simulink model "UAVIntegratedNavigationSystem"  (R2020b)
settings: Solver=FixedStepAuto  StartTime=0.0  StopTime=TFinal  FixedStep=IMUtime  RelTol=1e-3
values from neighbouring files (symbols this model uses):
  AIONtime = 1    [ModelSettings.m]
  BiasAccel = 9.81E-4    (= 0.000981)    [ModelSettings.m]
  BiasGyro = 2.424068405548E-4    (= 0.000242406840555)    [ModelSettings.m]
  CorrTimeOrientationGNSS = 1    [ModelSettings.m]
  CorrTimePositionGNSS = 1    [ModelSettings.m]
  CorrTimeVelocityGNSS = 1    [ModelSettings.m]
  delay = 1.5    [ModelSettings.m]
  e = 0.081819106    [ModelSettings.m]
  g0 = 9.780327    [ModelSettings.m]
  GNSStime = 0.2    [ModelSettings.m]
  H0 = 0.1    [ModelSettings.m]
  IMUtime = 0.01    [ModelSettings.m]
  indUAV = 2    [ModelSettings.m]
  LambdaInit = 0.6555    [ModelSettings.m]
  mass = 0.7    [ModelSettings.m]
  N = 100    [ModelSettings.m]
  PhiInit = 0.968    [ModelSettings.m]
  PitchDown = -PitchUp    (= -0.1)    [ModelSettings.m]
  PitchUp = 0.1    [ModelSettings.m]
  Ra = 6378.245    [ModelSettings.m]
  RollDown = -RollUp    (= -0.1)    [ModelSettings.m]
  RollUp = 0.1    [ModelSettings.m]
  SigmaAccel = 9.81E-4    (= 0.000981)    [ModelSettings.m]
  SigmaAION = 30    [ModelSettings.m]
  SigmaAltitudeGNSS = 3    [ModelSettings.m]
  SigmaGyro = 2.666475246102E-6    (= 2.6664752461e-06)    [ModelSettings.m]
  SigmaLaser = 5    [ModelSettings.m]
  SigmaOrientationGNSS = 0.00349    [ModelSettings.m]
  SigmaPositionGNSS = 1.5    [ModelSettings.m]
  SigmaVelocityGNSS = 0.03    [ModelSettings.m]
  SigmaVelocityUpGNSS = 0.03    [ModelSettings.m]
  U1down = 0    [ModelSettings.m]
  U1up = 4 * ForceCoeff * OmegaMax^2    (= 9.9858124)    [ModelSettings.m]
  U2down = -U2up    (= -2.4964531)    [ModelSettings.m]
  U2up = ForceCoeff * OmegaMax^2    (= 2.4964531)    [ModelSettings.m]
  U3down = -U3up    (= -2.4964531)    [ModelSettings.m]
  U3up = ForceCoeff * OmegaMax^2    (= 2.4964531)    [ModelSettings.m]
  U4down = -U4up    (= -0.2494604)    [ModelSettings.m]
  U4up = 2 * DragCoeff * OmegaMax^2    (= 0.2494604)    [ModelSettings.m]
  WEarth = 7.2921158553E-5    (= 7.2921158553e-05)    [ModelSettings.m]
undefined symbols (not defined in the file or in its folder): deg, Newton, rad, Raphson, s
libraries: simulink x11, sharedtransform x7, pid_lib x6, aerolibconvert2 x4, sharedutil x4
(part 1 of 5)
settings Model: Creator=Павел Ермаков  LastModifiedBy=Павел Ермаков

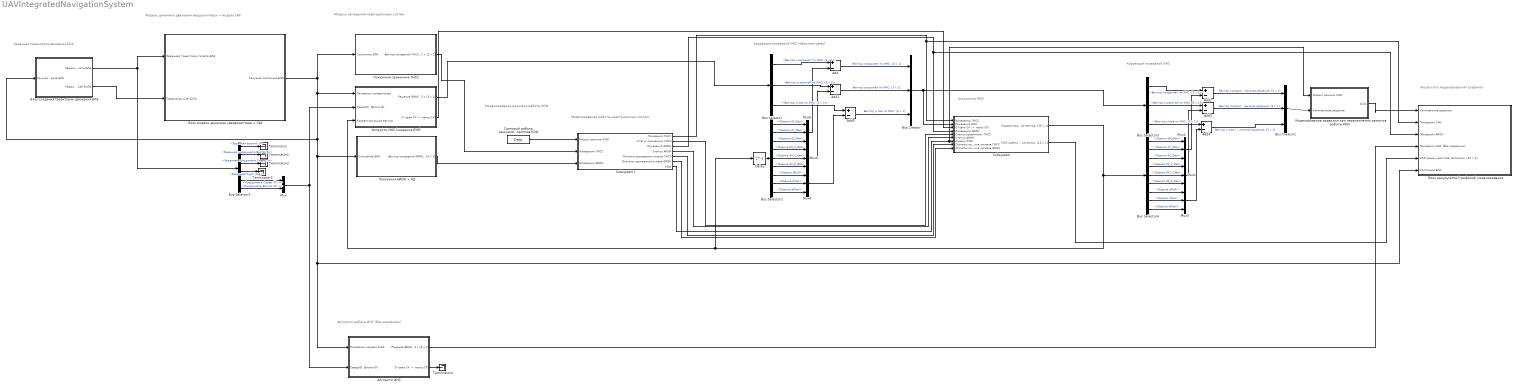
== system UAVIntegratedNavigationSystem ==
  note: Коррекция показаний ИНС (обратная связь)
  note: Модель измерений навигационных систем
  note: Модель динамики движения квадрокоптера + модель САУ
  note: Заданная траектория движения БЛА
  note: Коррекция показаний ИНС
  note: Результаты моделирования (графики)
  note: Алгоритмы КОИ
  note: Алгоритм работы ИНС (без коррекции)
  note: Моделирование режимоа работы КОИ
  note: Моделирование работы навигационных систем
  Add{,1..5} (6 alike) : Sum  Inputs=+-
  Bus Creator : BusCreator  Inputs=3
  Bus Creator1 : BusCreator  Inputs=3
  Bus Selector : BusSelector  OutputSignals=Вектор координат по ИНС; [3 x 1],Вектор скоростей по ИНС; [3 x 1],Вектор углов по ИНС; [3 x 1]
  Bus Selector1 : BusSelector  OutputSignals=Оценка dX_Geo,Оценка dY_Geo,Оценка dZ_Geo,Оценка dV_X_Geo,Оценка dV_Y_Geo,Оценка dV_Z_Geo,Оценка dRoll,Оценка dYaw,Оценка dPitch
  Bus Selector2 : BusSelector  OutputSignals=Заданная высота; м,Заданная координата Восток; м,Заданная координата Север; м,Заданный Курс; рад,Координата Север (0); м,Координата Восток (0); м
  Bus Selector3 : BusSelector  OutputSignals=Вектор координат по ИНС; [3 x 1],Вектор скорсотей по ИНС; [3 x 1],Вектор углов по ИНС; [3 x 1]
  Bus Selector4 : BusSelector  OutputSignals=Оценка dX_Geo,Оценка dY_Geo,Оценка dZ_Geo,Оценка dV_X_Geo,Оценка dV_Y_Geo,Оценка dV_Z_Geo,Оценка dRoll,Оценка dYaw,Оценка dPitch
  Delay : Delay  DelayLength=1  InitialCondition=0
  Mux : Mux  Inputs=2
  Mux{1..6} (6 alike) : Mux  Inputs=3
  Subsystem : Subsystem
  Subsystem1 : Subsystem
  Terminator{,1..4} (5 alike) : Terminator
  "Алгоритм ИНС " : Subsystem
      mask Display: image(imread('ins.jpg'))
  Алгоритм ИНС (коррекия БЧЭ) : Subsystem
      mask Display: image(imread('ins.jpg'))
  Блок модели динамики квадрокоптера + САУ : Subsystem
  Блок результатов (графиков) моделирования : Subsystem
  Блок создания траектории движения БЛА : Subsystem
  Моделирование задержки при переключении режимов работы КОИ : Subsystem
  Показания АИОН + ЛД : Subsystem
      mask Display: image(imread('Laser.jpg'))
  Показания приемника ГНСС : Subsystem
      mask Display: image(imread('satellite.jpg'))
  Сценарий работы режимов алгоритмов КОИ : FromWorkspace  VariableName=Data
  wires:
  Блок создания траектории движения БЛА/1(Заданная траектория полета БЛА) -> Bus Selector2/1, Блок модели динамики квадрокоптера + САУ/1(Заданная траектория полета БЛА)
  Bus Selector2/1 -> Terminator/1  "<Заданная высота; м>"
  Bus Selector2/2 -> Terminator1/1  "<Заданная координата Восток; м>"
  Bus Selector2/3 -> Terminator2/1  "<Заданная координата Север; м>"
  Bus Selector2/4 -> Terminator3/1  "<Заданный Курс; рад>"
  Bus Selector2/5 -> Mux/1  "<Координата Север (0); м>"
  Bus Selector2/6 -> Mux/2  "<Координата Восток (0); м>"
  Mux/1 -> "Алгоритм ИНС "/2("Север(0), Восток(0)"), Алгоритм ИНС (коррекия БЧЭ)/2("Север(0), Восток(0)")
  Алгоритм ИНС (коррекия БЧЭ)/1("Решение БИНС, 3 x [3 x 1]") -> Bus Selector/1
  Bus Selector1/5 -> Mux6/2  "<Оценка dV_Y_Geo>"
  Bus Selector1/4 -> Mux6/1  "<Оценка dV_X_Geo>"
  Bus Selector1/1 -> Mux5/1  "<Оценка dX_Geo>"
  Bus Selector1/2 -> Mux5/2  "<Оценка dY_Geo>"
  Bus Selector1/6 -> Mux6/3  "<Оценка dV_Z_Geo>"
  Bus Selector1/3 -> Mux5/3  "<Оценка dZ_Geo>"
  Bus Selector/1 -> Add/1  "<Вектор координат по ИНС; [3 x 1]>"
  Mux5/1 -> Add/2
  Bus Selector/2 -> Add1/1  "<Вектор скоростей по ИНС; [3 x 1]>"
  Mux6/1 -> Add1/2
  Add/1 -> Bus Creator/1  "Вектор координат по ИНС; [3 x 1]"
  Add1/1 -> Bus Creator/2  "Вектор скорсотей по ИНС; [3 x 1]"
  Bus Selector/3 -> Add5/1  "<Вектор углов по ИНС; [3 x 1]>"
  Bus Creator/1 -> Subsystem/2(Показания ИНС), Bus Selector3/1
  Delay/1 -> Bus Selector1/1
  Bus Selector3/1 -> Add2/1  "<Вектор координат по ИНС; [3 x 1]>"
  Bus Selector4/1 -> Mux1/1  "<Оценка dX_Geo>"
  Bus Selector4/2 -> Mux1/2  "<Оценка dY_Geo>"
  Bus Selector4/3 -> Mux1/3  "<Оценка dZ_Geo>"
  Mux1/1 -> Add2/2
  Bus Selector4/4 -> Mux2/1  "<Оценка dV_X_Geo>"
  Bus Selector4/5 -> Mux2/2  "<Оценка dV_Y_Geo>"
  Bus Selector4/6 -> Mux2/3  "<Оценка dV_Z_Geo>"
  Bus Selector3/2 -> Add3/1  "<Вектор скорсотей по ИНС; [3 x 1]>"
  Mux2/1 -> Add3/2
  Subsystem/1("Корректирующий вектор, [15 x 1]") -> Bus Selector4/1, Алгоритм ИНС (коррекия БЧЭ)/3(Корректирующий вектор), Delay/1
  Алгоритм ИНС (коррекия БЧЭ)/2("D (связ СК -> геогр СК)") -> Subsystem/3("D (связ СК -> геогр СК)")
  Add2/1 -> Bus Creator1/1  "Вектор координат комплексное решение; [3 x 1]"
  Add3/1 -> Bus Creator1/2  "Вектор скоростей комплексное решение; [3 x 1]"
  Bus Selector3/3 -> Add4/1  "<Вектор углов по ИНС; [3 x 1]>"
  Bus Creator1/1 -> Моделирование задержки при переключении режимов работы КОИ/2(Комплексное решение)
  Subsystem/2("СКО оценки вектора состояния, [15 x 1]") -> Блок результатов (графиков) моделирования/5("СКО оценки вектора состояния, [15 x 1]")
  Блок модели динамики квадрокоптера + САУ/1(Текущее состояние БЛА) -> Блок создания траектории движения БЛА/1(Текущее состояние БЛА), "Алгоритм ИНС "/1(Показания измерителей), Блок результатов (графиков) моделирования/6(Состояние БЛА), Показания АИОН + ЛД/1(Состояние БЛА), Алгоритм ИНС (коррекия БЧЭ)/1(Показания измерителей), Показания приемника ГНСС/1(Состояние БЛА)
  Add4/1 -> Bus Creator1/3  "Вектор углов комплексное решение; [3 x 1]"
  Bus Selector4/7 -> Mux3/1  "<Оценка dRoll>"
  Bus Selector4/9 -> Mux3/3  "<Оценка dPitch>"
  Bus Selector4/8 -> Mux3/2  "<Оценка dYaw>"
  Bus Selector1/7 -> Mux4/1  "<Оценка dRoll>"
  Bus Selector1/8 -> Mux4/2  "<Оценка dYaw>"
  Bus Selector1/9 -> Mux4/3  "<Оценка dPitch>"
  Add5/1 -> Bus Creator/3  "Вектор углов по ИНС; [3 x 1]"
  "Алгоритм ИНС "/2("D (связ СК -> геогр СК)") -> Terminator4/1
  "Алгоритм ИНС "/1("Решение БИНС, 3 x [3 x 1]") -> Блок результатов (графиков) моделирования/4(Показания ИНС (без коррекции))
  Mux3/1 -> Add4/2
  Показания АИОН + ЛД/1("Вектор измерений АИОН,  [3 x 1]") -> Subsystem1/3(Измерения АИОН)
  Показания приемника ГНСС/1("Вектор измерений ГНСС, 2 x [3 x 1]") -> Subsystem1/2(Измерения ГНСС)
  Subsystem1/1(Показания ГНСС) -> Subsystem/1(Измерения ГНСС), Блок результатов (графиков) моделирования/2(Показания СНС)
  Subsystem1/3(Показания АИОН) -> Subsystem/4(Измерения АИОН), Блок результатов (графиков) моделирования/3(Показания АИОН)
  Subsystem1/2(Статус применика ГНСС) -> Subsystem/5(Статус приемника  ГНСС)
  Subsystem1/4(Статус АИОН) -> Subsystem/6(Статус АИОН)
  Блок создания траектории движения БЛА/2(Параметры САУ БпЛА) -> Блок модели динамики квадрокоптера + САУ/2(Параметры САУ БпЛА)
  Subsystem1/6(Отсчеты пропадания сгнала АИОН) -> Subsystem/9(Отсчеты пропадания сигнала АИОН)
  Subsystem1/5(Отсчеты пропадания сгнала ГНСС) -> Subsystem/8(Отсчеты пропадания сигнала ГНСС)
  Subsystem1/7(КОИ) -> Subsystem/7(Индекс КОИ), Моделирование задержки при переключении режимов работы КОИ/1(Индекс режима КОИ)
  Mux4/1 -> Add5/2
  Моделирование задержки при переключении режимов работы КОИ/1(Out1) -> Блок результатов (графиков) моделирования/1(Комплексное решение)
  Сценарий работы режимов алгоритмов КОИ/1 -> Subsystem1/1(Индекс режима КОИ)

== system UAVIntegratedNavigationSystem/Subsystem ==
  Измерения ГНСС : Inport
  Показания ИНС : Inport  Port=2
  "D (связ СК -> геогр СК)" : Inport  Port=3
  Измерения АИОН : Inport  Port=4
  Статус приемника  ГНСС : Inport  Port=5
  Статус АИОН : Inport  Port=6
  Индекс КОИ : Inport  Port=7
  Отсчеты пропадания сигнала ГНСС : Inport  Port=8
  Отсчеты пропадания сигнала АИОН : Inport  Port=9
  Bus Creator2 : BusCreator  Inputs=15
  Bus Creator3 : BusCreator  Inputs=15
  Demux4 : Demux  Outputs=15
  Demux6 : Demux  Outputs=15
  MATLAB Function : MATLAB Function  TreatAsAtomicUnit=on
  MATLAB Function1 : MATLAB Function  TreatAsAtomicUnit=on
  Multiport Switch1 : MultiPortSwitch
  NaN : Constant  Value=NaN  OutDataTypeStr=Inherit: Inherit via back propagation
  Rate Transition : RateTransition  OutPortSampleTime=IMUtime
  Rate Transition1 : RateTransition  OutPortSampleTime=IMUtime
  Слабосвязанная схема комплексирования ИНС + АИОН : Subsystem
  Слабосвязанная схема комплексирования ИНС + ГНСС : Subsystem
  "Корректирующий вектор, [15 x 1]" : Outport
  "СКО оценки вектора состояния, [15 x 1]" : Outport  Port=2
  wires:
  "D (связ СК -> геогр СК)"/1 -> Слабосвязанная схема комплексирования ИНС + ГНСС/3("D (связ СК -> геогр СК)"), Слабосвязанная схема комплексирования ИНС + АИОН/3("D (связ СК -> геогр СК)")
  Слабосвязанная схема комплексирования ИНС + ГНСС/1("Корректирующий вектор, [15 x 1]") -> MATLAB Function1/3(INSGNSS), MATLAB Function/1(INSGNSS)
  Слабосвязанная схема комплексирования ИНС + ГНСС/2("СКО оценки вектора состояния, [15 x 1]") -> Multiport Switch1/2
  Demux4/14 -> Bus Creator2/14  "Оценка dGyroY"
  Demux4/10 -> Bus Creator2/10  "Оценка dAccX"
  Demux4/12 -> Bus Creator2/12  "Оценка dAccZ"
  Demux4/7 -> Bus Creator2/7  "Оценка dRoll"
  Demux4/6 -> Bus Creator2/6  "Оценка dV_Z_Geo"
  Demux4/8 -> Bus Creator2/8  "Оценка dYaw"
  Demux4/2 -> Bus Creator2/2  "Оценка dY_Geo"
  Demux4/3 -> Bus Creator2/3  "Оценка dZ_Geo"
  Demux4/9 -> Bus Creator2/9  "Оценка dPitch"
  Demux4/4 -> Bus Creator2/4  "Оценка dV_X_Geo"
  Demux4/1 -> Bus Creator2/1  "Оценка dX_Geo"
  Demux4/13 -> Bus Creator2/13  "Оценка dGyroX"
  Demux4/15 -> Bus Creator2/15  "Оценка dGyroZ"
  MATLAB Function/1(CorrectionVector) -> Demux4/1
  Demux4/11 -> Bus Creator2/11  "Оценка dAccY"
  Demux4/5 -> Bus Creator2/5  "Оценка dV_Y_Geo"
  Demux6/15 -> Bus Creator3/15  "СКО dGyroZ0"
  Bus Creator3/1 -> Rate Transition1/1
  Demux6/9 -> Bus Creator3/9  "СКО dPitch"
  Demux6/8 -> Bus Creator3/8  "СКО dYaw"
  Demux6/7 -> Bus Creator3/7  "СКО dRoll"
  Demux6/6 -> Bus Creator3/6  "СКО dVzGeo"
  Demux6/4 -> Bus Creator3/4  "СКО dVxGeo"
  Demux6/3 -> Bus Creator3/3  "СКО dZGeo"
  Demux6/5 -> Bus Creator3/5  "СКО dVyGeo"
  Demux6/2 -> Bus Creator3/2  "СКО dAltitude"
  Multiport Switch1/1 -> Demux6/1
  Demux6/11 -> Bus Creator3/11  "СКО dAccY0"
  Demux6/10 -> Bus Creator3/10  "СКО dAccX0"
  Demux6/13 -> Bus Creator3/13  "СКО dGyroX0"
  Demux6/14 -> Bus Creator3/14  "СКО dGyroY0"
  Demux6/1 -> Bus Creator3/1  "СКО dXGeo"
  Demux6/12 -> Bus Creator3/12  "СКО dAccZ0"
  Измерения ГНСС/1 -> Слабосвязанная схема комплексирования ИНС + ГНСС/2(Измерения ГНСС)
  Статус приемника  ГНСС/1 -> Слабосвязанная схема комплексирования ИНС + ГНСС/4(Статус приемника  ГНСС)
  Статус АИОН/1 -> Слабосвязанная схема комплексирования ИНС + АИОН/4(Статус АИОН)
  Слабосвязанная схема комплексирования ИНС + АИОН/2("СКО оценки вектора состояния, [15 x 1]") -> Multiport Switch1/3
  Слабосвязанная схема комплексирования ИНС + АИОН/1("Корректирующий вектор, [15 x 1]") -> MATLAB Function/2(INSAINS), MATLAB Function1/4(INSAINS)
  Измерения АИОН/1 -> Слабосвязанная схема комплексирования ИНС + АИОН/2(Измерения АИОН)
  NaN/1 -> Multiport Switch1/4
  Показания ИНС/1 -> Слабосвязанная схема комплексирования ИНС + ГНСС/1(Показания ИНС), Слабосвязанная схема комплексирования ИНС + АИОН/1(Показания ИНС)
  Bus Creator2/1 -> Rate Transition/1
  Индекс КОИ/1 -> MATLAB Function/4(indKOI), Multiport Switch1/1
  Отсчеты пропадания сигнала ГНСС/1 -> MATLAB Function1/1(SampleGNSSOff)
  Отсчеты пропадания сигнала АИОН/1 -> MATLAB Function1/2(SampleAINSOff)
  MATLAB Function1/1(y) -> MATLAB Function/3(INS)
  Rate Transition/1 -> "Корректирующий вектор, [15 x 1]"/1
  Rate Transition1/1 -> "СКО оценки вектора состояния, [15 x 1]"/1

== system UAVIntegratedNavigationSystem/Subsystem1 ==
  Индекс режима КОИ : Inport
  Измерения ГНСС : Inport  Port=2
  Измерения АИОН : Inport  Port=3
  Функционирование АИОН : Subsystem
  Функционирование приемника ГНСС : Subsystem
  Показания ГНСС : Outport
  Статус применика ГНСС : Outport  Port=2
  Показания АИОН : Outport  Port=3
  Статус АИОН : Outport  Port=4
  Отсчеты пропадания сгнала ГНСС : Outport  Port=5
  Отсчеты пропадания сгнала АИОН : Outport  Port=6
  КОИ : Outport  Port=7
  wires:
  Индекс режима КОИ/1 -> КОИ/1, Функционирование АИОН/1(КОИ), Функционирование приемника ГНСС/1(КОИ)
  Функционирование приемника ГНСС/1(Измерения приемника ГНСС (выход)) -> Показания ГНСС/1
  Измерения ГНСС/1 -> Функционирование приемника ГНСС/2(Измерения приемника ГНСС)
  Функционирование приемника ГНСС/2(Статус приемника (-1/0 / 1)) -> Статус применика ГНСС/1
  Функционирование АИОН/1(Измерения АИОН (выход)) -> Показания АИОН/1
  Функционирование АИОН/2(Статус АИОН (-1/0 / 1)) -> Статус АИОН/1
  Измерения АИОН/1 -> Функционирование АИОН/2(Измерения АИОН)
  Функционирование приемника ГНСС/3(Количество отсчетов после проадания сигнала ГНСС) -> Отсчеты пропадания сгнала ГНСС/1
  Функционирование АИОН/3(Количество отсчетов после проадания сигнала АИОН) -> Отсчеты пропадания сгнала АИОН/1

== system UAVIntegratedNavigationSystem/Алгоритм ИНС  ==
  Показания измерителей : Inport
  "Север(0), Восток(0)" : Inport  Port=2
  Bus Creator : BusCreator  Inputs=5
  Bus Selector : BusSelector  OutputSignals=AngX,AngY,AngZ,AccX,AccY,AccZ
  Demux : Demux  Outputs=2
  Matrix Multiply : Product  Multiplication=Matrix(*)
  Matrix Multiply1 : Product  Multiplication=Matrix(*)
  Mux : Mux  Inputs=3
  Mux1 : Mux  Inputs=3
  Transpose : Math  Operator=transpose  SaturateOnIntegerOverflow=on
  Алгоритм Навигации : Subsystem
  Алгоритм Ориентации : Subsystem
  Блок ошибок ДУС : Subsystem
  Блок ошибок акселерометров : Subsystem
  Блок пересчета : Subsystem
  Вычисление углов : Subsystem
  "Решение БИНС, 3 x [3 x 1]" : Outport  SampleTime=IMUtime
  "D (связ СК -> геогр СК)" : Outport  Port=2  SampleTime=IMUtime
  wires:
  Показания измерителей/1 -> Bus Selector/1
  Алгоритм Навигации/2(OmegaG) -> Алгоритм Ориентации/2(OmegaG)  "WG"
  Алгоритм Навигации/1("Координаты, скорости БЛА") -> Demux/1
  Bus Creator/1 -> "Решение БИНС, 3 x [3 x 1]"/1
  Алгоритм Ориентации/1("Матрица перевода D(связ СК -> геогр СК)") -> Matrix Multiply1/1, Matrix Multiply1/2, "D (связ СК -> геогр СК)"/1, Вычисление углов/1("D (связ СК -> геогр СК)"), Блок пересчета/1("D (связ СК -> геогр СК)"), Transpose/1  "D (связ СК -> геогр СК)"
  Вычисление углов/1(Углы ориентации) -> Bus Creator/3  "Вектор углов по ИНС, [3 x 1]"
  Блок пересчета/1(Показания акселерометров (геогр СК)) -> Bus Creator/4, Алгоритм Навигации/1(Показания акселерометров (геогр СК))  "Вектор показаний акселерометров (геогр СК), [3 x 1]"
  Bus Selector/1 -> Mux/1  "<AngX>"
  Bus Selector/2 -> Mux/2  "<AngY>"
  Bus Selector/3 -> Mux/3  "<AngZ>"
  Bus Selector/4 -> Mux1/1  "<AccX>"
  Bus Selector/5 -> Mux1/2  "<AccY>"
  Bus Selector/6 -> Mux1/3  "<AccZ>"
  Mux1/1 -> Matrix Multiply/2
  Transpose/1 -> Matrix Multiply/1
  "Север(0), Восток(0)"/1 -> Алгоритм Навигации/2("Север(0), Восток(0)")
  Demux/1 -> Bus Creator/1  "Вектор координат по ИНС, [3 x 1]"
  Demux/2 -> Bus Creator/2  "Вектор скоростей по ИНС, [3 x 1]"
  Mux/1 -> Блок ошибок ДУС/1(Истинные значения)
  Matrix Multiply/1 -> Блок ошибок акселерометров/1(Истинные значения)
  Блок ошибок акселерометров/1(Показания акселерометров) -> Блок пересчета/2(Показания акселерометров (связ СК))
  Matrix Multiply1/1 -> Bus Creator/5  "Вектор показаний ДУСов (геогр. СК), [3x1]"
  Блок ошибок ДУС/1(Показания ДУС) -> Алгоритм Ориентации/1(Показания ДУС (связ СК))

== system UAVIntegratedNavigationSystem/Алгоритм ИНС (коррекия БЧЭ) ==
  Показания измерителей : Inport
  "Север(0), Восток(0)" : Inport  Port=2
  Корректирующий вектор : Inport  Port=3
  Add : Sum  Inputs=+-
  Add1 : Sum  Inputs=+-
  Bus Creator : BusCreator  Inputs=3
  Bus Selector : BusSelector  OutputSignals=AngX,AngY,AngZ,AccX,AccY,AccZ
  Bus Selector1 : BusSelector  OutputSignals=Оценка dAccX,Оценка dAccY,Оценка dAccZ,Оценка dGyroX,Оценка dGyroY,Оценка dGyroZ
  Delay : Delay  DelayLength=1  InitialCondition=0
  Demux : Demux  Outputs=2
  Matrix Multiply : Product  Multiplication=Matrix(*)
  Mux{,1,4..5} (4 alike) : Mux  Inputs=3
  Transpose : Math  Operator=transpose  SaturateOnIntegerOverflow=on
  Алгоритм Навигации : Subsystem
  Алгоритм Ориентации : Subsystem
  Блок ошибок ДУС : Subsystem
  Блок ошибок акселерометров : Subsystem
  Блок пересчета : Subsystem
  Вычисление углов : Subsystem
  "Решение БИНС, 3 x [3 x 1]" : Outport  SampleTime=IMUtime
  "D (связ СК -> геогр СК)" : Outport  Port=2  SampleTime=IMUtime
  wires:
  Показания измерителей/1 -> Bus Selector/1
  Алгоритм Навигации/2(OmegaG) -> Алгоритм Ориентации/2(OmegaG)  "WG"
  Алгоритм Навигации/1("Координаты, скорости БЛА") -> Demux/1
  Bus Creator/1 -> "Решение БИНС, 3 x [3 x 1]"/1
  Алгоритм Ориентации/1("Матрица перевода D(связ СК -> геогр СК)") -> "D (связ СК -> геогр СК)"/1, Вычисление углов/1("D (связ СК -> геогр СК)"), Блок пересчета/1("D (связ СК -> геогр СК)"), Transpose/1  "D (связ СК -> геогр СК)"
  Вычисление углов/1(Углы ориентации) -> Bus Creator/3  "Вектор углов по ИНС, [3 x 1]"
  Блок пересчета/1(Показания акселерометров (геогр СК)) -> Алгоритм Навигации/1(Показания акселерометров (геогр СК))  "Вектор показаний акселерометров (геогр СК), [3 x 1]"
  Bus Selector/1 -> Mux/1  "<AngX>"
  Bus Selector/2 -> Mux/2  "<AngY>"
  Bus Selector/3 -> Mux/3  "<AngZ>"
  Bus Selector/4 -> Mux1/1  "<AccX>"
  Bus Selector/5 -> Mux1/2  "<AccY>"
  Bus Selector/6 -> Mux1/3  "<AccZ>"
  Mux1/1 -> Matrix Multiply/2
  Transpose/1 -> Matrix Multiply/1
  "Север(0), Восток(0)"/1 -> Алгоритм Навигации/2("Север(0), Восток(0)")
  Demux/1 -> Bus Creator/1  "Вектор координат по ИНС, [3 x 1]"
  Demux/2 -> Bus Creator/2  "Вектор скоростей по ИНС, [3 x 1]"
  Mux/1 -> Блок ошибок ДУС/1(Истинные значения)
  Блок ошибок ДУС/1(Показания ДУС) -> Add1/1
  Matrix Multiply/1 -> Блок ошибок акселерометров/1(Истинные значения)
  Блок ошибок акселерометров/1(Показания акселерометров) -> Add/1
  Корректирующий вектор/1 -> Delay/1
  Delay/1 -> Bus Selector1/1
  Add/1 -> Блок пересчета/2(Показания акселерометров (связ СК))
  Bus Selector1/1 -> Mux4/1  "<Оценка dAccX>"
  Bus Selector1/2 -> Mux4/2  "<Оценка dAccY>"
  Bus Selector1/3 -> Mux4/3  "<Оценка dAccZ>"
  Mux4/1 -> Add/2
  Add1/1 -> Алгоритм Ориентации/1(Показания ДУС (связ СК))
  Bus Selector1/4 -> Mux5/1  "<Оценка dGyroX>"
  Bus Selector1/6 -> Mux5/3  "<Оценка dGyroZ>"
  Bus Selector1/5 -> Mux5/2  "<Оценка dGyroY>"
  Mux5/1 -> Add1/2

== system UAVIntegratedNavigationSystem/Блок модели динамики квадрокоптера + САУ ==
  Заданная траектория полета БЛА : Inport
  Параметры САУ БпЛА : Inport  Port=2
  Bus Selector : BusSelector  OutputSignals=Y,Z,X
  Bus Selector1 : BusSelector  OutputSignals=Pitch,Psi,Roll
  Bus Selector2 : BusSelector  OutputSignals=Заданная высота; м,Заданная координата Восток; м,Заданная координата Север; м,Заданный Курс; рад,Координата Север (0); м,Координата Восток (0); м
  Mux : Mux  Inputs=2
  Полетный контроллер : Subsystem
      mask Display: image(imread('controller.jpg'))
  "Упрощенная динамика БЛА " : Subsystem
      mask Display: image(imread('quadcopter.jpg'))
  Ускорение силы тяжести на широте phi : Subsystem
  Текущее состояние БЛА : Outport
  wires:
  Bus Selector/1 -> Полетный контроллер/5(<Y>)  "<Y>"
  Bus Selector/3 -> Полетный контроллер/7(<X>)  "<X>"
  Ускорение силы тяжести на широте phi/1(g(phi)) -> "Упрощенная динамика БЛА "/2(g), Полетный контроллер/11(g)
  Bus Selector/2 -> Полетный контроллер/6(<Z>)  "<Z>"
  Bus Selector1/2 -> Полетный контроллер/9(<Psi>)  "<Psi>"
  Bus Selector1/3 -> Полетный контроллер/8(<Roll>)  "<Roll>"
  "Упрощенная динамика БЛА "/1(Состояние БЛА) -> Ускорение силы тяжести на широте phi/1("(X, Y, Z, ph)i"), Bus Selector1/1, Текущее состояние БЛА/1, Bus Selector/1
  Bus Selector1/1 -> Полетный контроллер/10(<Pitch>)  "<Pitch>"
  Заданная траектория полета БЛА/1 -> Bus Selector2/1
  Bus Selector2/1 -> Полетный контроллер/1(Высота заданная)  "<Заданная высота; м>"
  Bus Selector2/2 -> Полетный контроллер/2("  Z заданная")  "<Заданная координата Восток; м>"
  Bus Selector2/3 -> Полетный контроллер/3(X заданная)  "<Заданная координата Север; м>"
  Bus Selector2/4 -> Полетный контроллер/4(Курс заданный)  "<Заданный Курс; рад>"
  Bus Selector2/5 -> Mux/1  "<Координата Север (0); м>"
  Bus Selector2/6 -> Mux/2  "<Координата Восток (0); м>"
  Полетный контроллер/1(U1) -> "Упрощенная динамика БЛА "/1(U1)
  Mux/1 -> "Упрощенная динамика БЛА "/3("Север(0), Восток(0)")
  Полетный контроллер/2(U2) -> "Упрощенная динамика БЛА "/4(U2)
  Полетный контроллер/3(U3) -> "Упрощенная динамика БЛА "/5(U3)
  Полетный контроллер/4(U4) -> "Упрощенная динамика БЛА "/6(U4)
  Параметры САУ БпЛА/1 -> Полетный контроллер/12(Параметры САУ БпЛА)

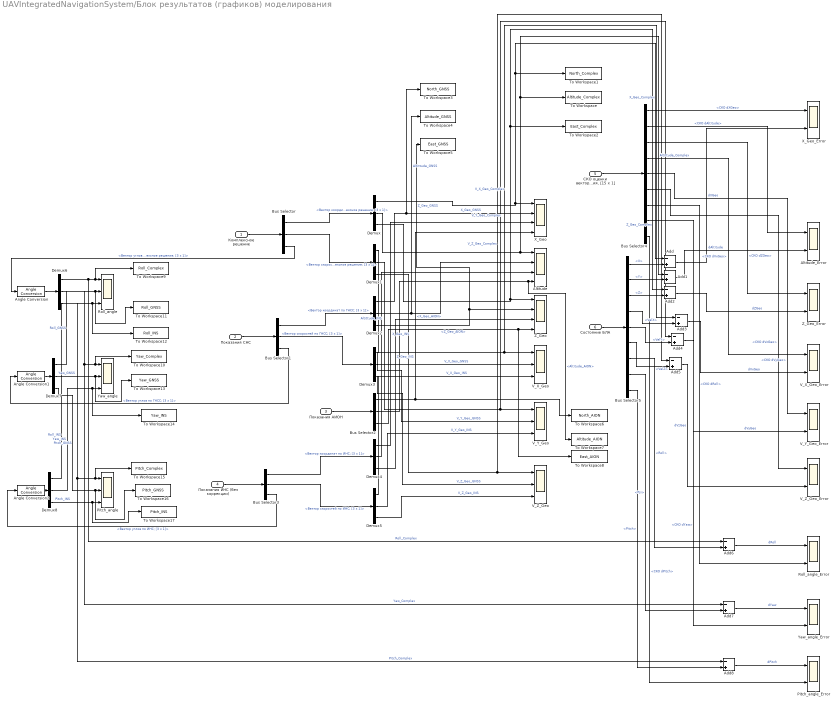
== system UAVIntegratedNavigationSystem/Блок результатов (графиков) моделирования ==
  Комплексное решение : Inport
  Показания СНС : Inport  Port=2
  Показания АИОН : Inport  Port=3
  Показания ИНС (без коррекции) : Inport  Port=4
  "СКО оценки вектора состояния, [15 x 1]" : Inport  Port=5
  Состояние БЛА : Inport  Port=6
  Add{,1..8} (9 alike) : Sum  Inputs=-+
  Altitude : Scope  NumInputPorts=4
  Altitude_Error : Scope  NumInputPorts=2
  Angle Conversion : aerolibconvert2/Angle Conversion  IU=rad  OU=deg
  Angle Conversion1 : aerolibconvert2/Angle Conversion  IU=rad  OU=deg
  Angle Conversion2 : aerolibconvert2/Angle Conversion  IU=rad  OU=deg
  Bus Selector : BusSelector  OutputSignals=Вектор координат комплексное решение; [3 x 1],Вектор скоростей комплексное решение; [3 x 1],Вектор углов комплексное решение; [3 x 1]
  Bus Selector1 : BusSelector  OutputSignals=Вектор координат по ГНСС; [3 x 1],Вектор скоростей по ГНСС; [3 x 1],Вектор углов по ГНСС; [3 x 1]
  Bus Selector2 : BusSelector  OutputSignals=X_Geo_AION,Altitude_AION,Z_Geo_AION
  Bus Selector3 : BusSelector  OutputSignals=Вектор координат по ИНС; [3 x 1],Вектор скоростей по ИНС; [3 x 1],Вектор углов по ИНС; [3 x 1]
  Bus Selector4 : BusSelector  OutputSignals=СКО dXGeo,СКО dAltitude,СКО dZGeo,СКО dVxGeo,СКО dVyGeo,СКО dVzGeo,СКО dRoll,СКО dYaw,СКО dPitch
  Bus Selector5 : BusSelector  OutputSignals=X,Y,Z,VelX,VelY,VelZ,Roll,Psi,Pitch
  Demux{,1..8} (9 alike) : Demux  Outputs=3
  Pitch_angle : Scope  NumInputPorts=3
  Pitch_angle_Error : Scope  NumInputPorts=2
  Roll_angle : Scope  NumInputPorts=3
  Roll_angle_Error : Scope  NumInputPorts=2
  To Workspace : ToWorkspace  VariableName=Altitude_Complex  SaveFormat=Timeseries  SampleTime=IMUtime
  To Workspace1 : ToWorkspace  VariableName=North_Complex  SaveFormat=Timeseries  SampleTime=IMUtime
  To Workspace10 : ToWorkspace  VariableName=Yaw_Complex  SaveFormat=Timeseries  SampleTime=IMUtime
  To Workspace11 : ToWorkspace  VariableName=Roll_GNSS  SaveFormat=Timeseries  SampleTime=GNSStime
  To Workspace12 : ToWorkspace  VariableName=Roll_INS  SaveFormat=Timeseries  SampleTime=IMUtime
  To Workspace13 : ToWorkspace  VariableName=Yaw_GNSS  SaveFormat=Timeseries  SampleTime=GNSStime
  To Workspace14 : ToWorkspace  VariableName=Yaw_INS  SaveFormat=Timeseries  SampleTime=IMUtime
  To Workspace15 : ToWorkspace  VariableName=Pitch_Complex  SaveFormat=Timeseries  SampleTime=IMUtime
  To Workspace16 : ToWorkspace  VariableName=Pitch_GNSS  SaveFormat=Timeseries  SampleTime=GNSStime
  To Workspace17 : ToWorkspace  VariableName=Pitch_INS  SaveFormat=Timeseries  SampleTime=IMUtime
  To Workspace2 : ToWorkspace  VariableName=East_Complex  SaveFormat=Timeseries  SampleTime=IMUtime
  To Workspace3 : ToWorkspace  VariableName=North_GNSS  SaveFormat=Timeseries  SampleTime=GNSStime
  To Workspace4 : ToWorkspace  VariableName=Altitude_GNSS  SaveFormat=Timeseries  SampleTime=GNSStime
  To Workspace5 : ToWorkspace  VariableName=East_GNSS  SaveFormat=Timeseries  SampleTime=GNSStime
  To Workspace6 : ToWorkspace  VariableName=North_AION  SaveFormat=Timeseries  SampleTime=AIONtime
  To Workspace7 : ToWorkspace  VariableName=Altitude_AION  SaveFormat=Timeseries  SampleTime=AIONtime
  To Workspace8 : ToWorkspace  VariableName=East_AION  SaveFormat=Timeseries  SampleTime=AIONtime
  To Workspace9 : ToWorkspace  VariableName=Roll_Complex  SaveFormat=Timeseries  SampleTime=IMUtime
  V_X_Geo : Scope  NumInputPorts=3
  V_X_Geo_Error : Scope  NumInputPorts=2
  V_Y_Geo : Scope  NumInputPorts=3
  V_Y_Geo_Error : Scope  NumInputPorts=2
  V_Z_Geo : Scope  NumInputPorts=3
  V_Z_Geo_Error : Scope  NumInputPorts=2
  X_Geo : Scope  NumInputPorts=4
  X_Geo_Error : Scope  NumInputPorts=2
  Yaw_angle : Scope  NumInputPorts=3
  Yaw_angle_Error : Scope  NumInputPorts=2
  Z_Geo : Scope  NumInputPorts=4
  Z_Geo_Error : Scope  NumInputPorts=2
  wires:
  Комплексное решение/1 -> Bus Selector/1
  Показания СНС/1 -> Bus Selector1/1
  Показания АИОН/1 -> Bus Selector2/1
  Показания ИНС (без коррекции)/1 -> Bus Selector3/1
  Bus Selector/1 -> Demux/1  "<Вектор координат комплексное решение; [3 x 1]>"
  Bus Selector/2 -> Demux1/1  "<Вектор скоростей комплексное решение; [3 x 1]>"
  Bus Selector1/1 -> Demux2/1  "<Вектор координат по ГНСС; [3 x 1]>"
  Bus Selector3/1 -> Demux4/1  "<Вектор координат по ИНС; [3 x 1]>"
  Demux4/1 -> X_Geo/3  "X_Geo_INS"
  Demux4/2 -> Altitude/3  "Altittude_INS"
  Demux4/3 -> Z_Geo/3  "Z_Geo_INS"
  Bus Selector3/2 -> Demux5/1  "<Вектор скоростей по ИНС; [3 x 1]>"
  Demux5/2 -> V_Y_Geo/3  "V_Y_Geo_INS"
  Demux5/1 -> V_X_Geo/3  "V_X_Geo_INS"
  Demux5/3 -> V_Z_Geo/3  "V_Z_Geo_INS"
  Demux/1 -> Add/1, To Workspace1/1, X_Geo/1  "X_Geo_Complex"
  Demux2/1 -> To Workspace3/1, X_Geo/2  "X_Geo_GNSS"
  Demux/2 -> Add1/1, To Workspace/1, Altitude/1  "Altittude_Complex"
  Demux2/2 -> Altitude/2, To Workspace4/1  "Altittude_GNSS"
  Demux/3 -> Add2/1, To Workspace2/1, Z_Geo/1  "Z_Geo_Complex"
  Demux2/3 -> To Workspace5/1, Z_Geo/2  "Z_Geo_GNSS"
  Demux1/1 -> V_X_Geo/1, Add3/1  "V_X_Geo_Complex"
  Demux3/1 -> V_X_Geo/2  "V_X_Geo_GNSS"
  Demux1/2 -> Add4/1, V_Y_Geo/1  "V_Y_Geo_Complex"
  Demux3/2 -> V_Y_Geo/2  "V_Y_Geo_GNSS"
  Demux3/3 -> V_Z_Geo/2  "V_Z_Geo_GNSS"
  Demux1/3 -> V_Z_Geo/1, Add5/1  "V_Z_Geo_Complex"
  "СКО оценки вектора состояния, [15 x 1]"/1 -> Bus Selector4/1
  Состояние БЛА/1 -> Bus Selector5/1
  Bus Selector4/1 -> X_Geo_Error/1  "<СКО dXGeo>"
  Add/1 -> X_Geo_Error/2  "dXGeo"
  Bus Selector5/1 -> Add/2  "<X>"
  Bus Selector4/2 -> Altitude_Error/1  "<СКО dAltitude>"
  Bus Selector5/2 -> Add1/2  "<Y>"
  Add1/1 -> Altitude_Error/2  "dAltitude"
  Bus Selector4/3 -> Z_Geo_Error/1  "<СКО dZGeo>"
  Bus Selector5/3 -> Add2/2  "<Z>"
  Add2/1 -> Z_Geo_Error/2  "dZGeo"
  Bus Selector4/4 -> V_X_Geo_Error/1  "<СКО dVxGeo>"
  Bus Selector5/4 -> Add3/2  "<VelX>"
  Add3/1 -> V_X_Geo_Error/2  "dVxGeo"
  Bus Selector5/5 -> Add4/2  "<VelY>"
  Add4/1 -> V_Y_Geo_Error/2  "dVyGeo"
  Bus Selector4/5 -> V_Y_Geo_Error/1  "<СКО dVyGeo>"
  Bus Selector5/6 -> Add5/2  "<VelZ>"
  Add5/1 -> V_Z_Geo_Error/2  "dVzGeo"
  Bus Selector4/6 -> V_Z_Geo_Error/1  "<СКО dVzGeo>"
  Bus Selector/3 -> Angle Conversion/1  "<Вектор углов комплексное решение; [3 x 1]>"
  Bus Selector1/3 -> Angle Conversion1/1  "<Вектор углов по ГНСС; [3 x 1]>"
  Bus Selector3/3 -> Angle Conversion2/1  "<Вектор углов по ИНС; [3 x 1]>"
  Demux6/1 -> To Workspace9/1, Roll_angle/1, Add6/1  "Roll_Complex"
  Demux7/1 -> To Workspace11/1, Roll_angle/2  "Roll_GNSS"
  Demux8/1 -> Roll_angle/3, To Workspace12/1  "Roll_INS"
  Demux6/2 -> Add7/1, To Workspace10/1, Yaw_angle/1  "Yaw_Complex"
  Demux7/2 -> To Workspace13/1, Yaw_angle/2  "Yaw_GNSS"
  Demux8/2 -> Yaw_angle/3, To Workspace14/1  "Yaw_INS"
  Demux8/3 -> Pitch_angle/3, To Workspace17/1  "Pitch_INS"
  Demux7/3 -> To Workspace16/1, Pitch_angle/2  "Pitch_GNSS"
  Demux6/3 -> To Workspace15/1, Pitch_angle/1, Add8/1  "Pitch_Complex"
  Add6/1 -> Roll_angle_Error/1  "dRoll"
  Bus Selector5/7 -> Add6/2  "<Roll>"
  Bus Selector4/7 -> Roll_angle_Error/2  "<СКО dRoll>"
  Add7/1 -> Yaw_angle_Error/1  "dYaw"
  Bus Selector4/8 -> Yaw_angle_Error/2  "<СКО dYaw>"
  Add8/1 -> Pitch_angle_Error/1  "dPitch"
  Bus Selector5/8 -> Add7/2  "<Psi>"
  Bus Selector5/9 -> Add8/2  "<Pitch>"
  Bus Selector4/9 -> Pitch_angle_Error/2  "<СКО dPitch>"
  Bus Selector2/1 -> To Workspace6/1, X_Geo/4  "<X_Geo_AION>"
  Bus Selector2/2 -> To Workspace7/1, Altitude/4  "<Altitude_AION>"
  Bus Selector2/3 -> Z_Geo/4, To Workspace8/1  "<Z_Geo_AION>"
  Bus Selector1/2 -> Demux3/1  "<Вектор скоростей по ГНСС; [3 x 1]>"
  Angle Conversion/1 -> Demux6/1
  Angle Conversion1/1 -> Demux7/1
  Angle Conversion2/1 -> Demux8/1

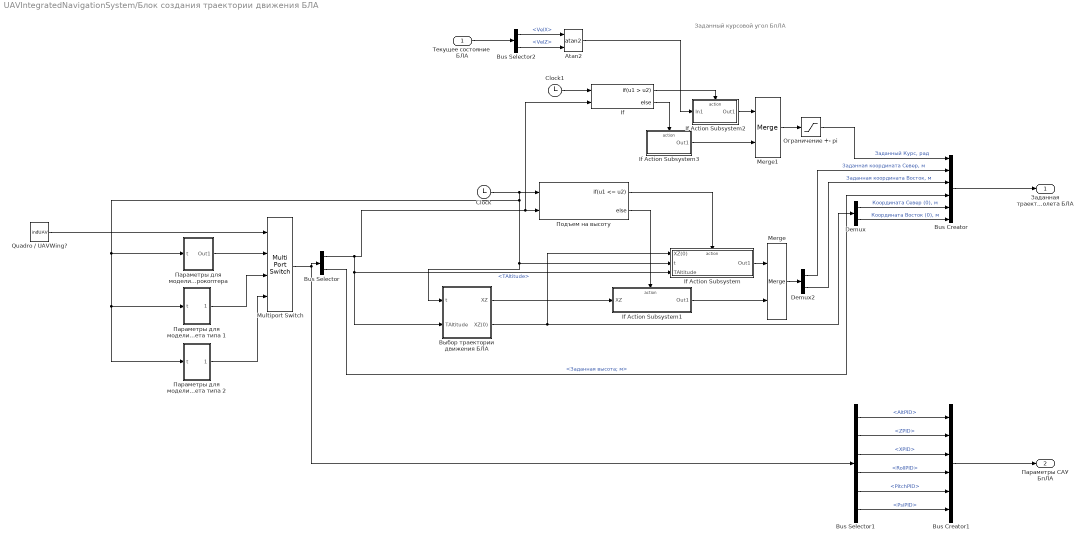
== system UAVIntegratedNavigationSystem/Блок создания траектории движения БЛА ==
  note: Заданный курсовой угол БпЛА
  Текущее состояние БЛА : Inport
  Atan2 : Trigonometry  Operator=atan2
  Bus Creator : BusCreator  Inputs=6
  Bus Creator1 : BusCreator  Inputs=6
  Bus Selector : BusSelector  OutputSignals=TAltitude,Заданная высота; м
  Bus Selector1 : BusSelector  OutputSignals=AltPID,ZPID,XPID,RollPID,PitchPID,PsiPID
  Bus Selector2 : BusSelector  OutputSignals=VelX,VelZ
  Clock : Clock
  Clock1 : Clock
  Demux : Demux  Outputs=2
  Demux2 : Demux  Outputs=2
  If : If  NumInputs=2  IfExpression=u1 > u2
  If Action Subsystem : Subsystem  TreatAsAtomicUnit=on
  If Action Subsystem1 : Subsystem  TreatAsAtomicUnit=on
  If Action Subsystem2 : Subsystem  TreatAsAtomicUnit=on
  If Action Subsystem3 : Subsystem  TreatAsAtomicUnit=on
  Merge : Merge
  Merge1 : Merge
  Multiport Switch : MultiPortSwitch
  Quadro / UAVWing? : Constant  Value=indUAV
  Выбор траектории движения БЛА : Subsystem
  Ограничение +- pi : Saturate  UpperLimit=pi  LowerLimit=-pi
  Параметры для моделирования самолета типа 1 : Subsystem
  Параметры для моделирования самолета типа 2 : Subsystem
  Параметры для моделирования квадрокоптера : Subsystem
  Подъем на высоту : If  NumInputs=2  IfExpression=u1 <= u2
  Заданная траектория полета БЛА : Outport
  Параметры САУ БпЛА : Outport  Port=2
  wires:
  If Action Subsystem1/1(Out1) -> Merge/2
  If Action Subsystem/1(Out1) -> Merge/1
  Clock/1 -> Выбор траектории движения БЛА/1(t), If Action Subsystem/2(t), Параметры для моделирования самолета типа 1/1(t), Параметры для моделирования самолета типа 2/1(t), Параметры для моделирования квадрокоптера/1(t), Подъем на высоту/1
  Подъем на высоту/2 -> If Action Subsystem1/Action
  Подъем на высоту/1 -> If Action Subsystem/Action
  Demux2/2 -> Bus Creator/3  "Заданная координата Восток, м"
  Merge/1 -> Demux2/1
  Demux2/1 -> Bus Creator/2  "Заданная координата Север, м"
  Merge1/1 -> Ограничение +- pi/1
  Bus Creator/1 -> Заданная траектория полета БЛА/1
  Выбор траектории движения БЛА/1(XZ) -> If Action Subsystem1/1(XZ)
  Выбор траектории движения БЛА/2(XZ(0)) -> If Action Subsystem/1(XZ(0)), Demux/1
  Demux/1 -> Bus Creator/5  "Координата Север (0), м"
  Demux/2 -> Bus Creator/6  "Координата Восток (0), м"
  Quadro / UAVWing?/1 -> Multiport Switch/1
  Multiport Switch/1 -> Bus Selector/1, Bus Selector1/1
  Bus Selector/1 -> Подъем на высоту/2, If/2, Выбор траектории движения БЛА/2(TAltitude), If Action Subsystem/3(TAltitude)  "<TAltitude>"
  Параметры для моделирования квадрокоптера/1(Out1) -> Multiport Switch/2
  Bus Selector/2 -> Bus Creator/4  "<Заданная высота; м>"
  Bus Creator1/1 -> Параметры САУ БпЛА/1
  Bus Selector1/1 -> Bus Creator1/1  "<AltPID>"
  Bus Selector1/6 -> Bus Creator1/6  "<PsiPID>"
  Bus Selector1/2 -> Bus Creator1/2  "<ZPID>"
  Bus Selector1/3 -> Bus Creator1/3  "<XPID>"
  Bus Selector1/4 -> Bus Creator1/4  "<RollPID>"
  Bus Selector1/5 -> Bus Creator1/5  "<PitchPID>"
  Текущее состояние БЛА/1 -> Bus Selector2/1
  Bus Selector2/1 -> Atan2/1  "<VelX>"
  Bus Selector2/2 -> Atan2/2  "<VelZ>"
  Clock1/1 -> If/1
  If/1 -> If Action Subsystem2/Action
  Atan2/1 -> If Action Subsystem2/1(In1)
  If/2 -> If Action Subsystem3/Action
  If Action Subsystem2/1(Out1) -> Merge1/1
  If Action Subsystem3/1(Out1) -> Merge1/2
  Ограничение +- pi/1 -> Bus Creator/1  "Заданный Курс, рад"
  Параметры для моделирования самолета типа 1/1(Out1) -> Multiport Switch/3
  Параметры для моделирования самолета типа 2/1(Out1) -> Multiport Switch/4

== system UAVIntegratedNavigationSystem/Моделирование задержки при переключении режимов работы КОИ ==
  note: Моделирование задержки при переключении режимов КОИ во избежание всплесков фильтра
  Индекс режима КОИ : Inport
  Комплексное решение : Inport  Port=2
  Add9 : Sum  Inputs=+-
  Clock : Clock
  Delay1 : Delay  DelayLength=delay/IMUtime  InitialCondition=0  SampleTime=IMUtime
  If : If  IfExpression=u1 ~= 0
  If Action Subsystem : Subsystem  TreatAsAtomicUnit=on
  If Action Subsystem1 : Subsystem  TreatAsAtomicUnit=on
  If Action Subsystem2 : Subsystem  TreatAsAtomicUnit=on
  If Action Subsystem3 : Subsystem  TreatAsAtomicUnit=on
  If1 : If  IfExpression=u1 > delay
  Memory : Memory
  Merge : Merge
  Merge1 : Merge
  Out1 : Outport
  wires:
  Merge1/1 -> Add9/2
  If1/1 -> If Action Subsystem2/Action
  If Action Subsystem3/1(Out1) -> Merge1/2
  Add9/1 -> If/1
  If1/2 -> If Action Subsystem3/Action
  Delay1/1 -> If Action Subsystem2/1(In1)
  Clock/1 -> If1/1
  Индекс режима КОИ/1 -> Add9/1, If Action Subsystem3/1(KOI), Delay1/1
  If/2 -> If Action Subsystem1/Action
  Memory/1 -> If Action Subsystem/1(In1)
  If/1 -> If Action Subsystem/Action
  If Action Subsystem1/1(Out1) -> Merge/2
  If Action Subsystem2/1(Out1) -> Merge1/1
  Merge/1 -> Out1/1, Memory/1
  If Action Subsystem/1(Out1) -> Merge/1
  Комплексное решение/1 -> If Action Subsystem1/1(Индекс режима КОИ)

== system UAVIntegratedNavigationSystem/Показания АИОН + ЛД ==
  Состояние БЛА : Inport
  Измерения АИОН + ЛД : Subsystem
  "Вектор измерений АИОН,  [3 x 1]" : Outport  SampleTime=AIONtime
  wires:
  Состояние БЛА/1 -> Измерения АИОН + ЛД/1("Состояние БЛА ")
  Измерения АИОН + ЛД/1("Измерения АИОН + ЛД,  [3 x 1]") -> "Вектор измерений АИОН,  [3 x 1]"/1

== system UAVIntegratedNavigationSystem/Показания приемника ГНСС ==
  Состояние БЛА : Inport
  Измерения ГНСС : Subsystem
  "Вектор измерений ГНСС, 2 x [3 x 1]" : Outport  SampleTime=GNSStime
  wires:
  Состояние БЛА/1 -> Измерения ГНСС/1("Состояние БЛА ")
  Измерения ГНСС/1("Измерения приемника ГНСС, 2 x [3 x 1]") -> "Вектор измерений ГНСС, 2 x [3 x 1]"/1

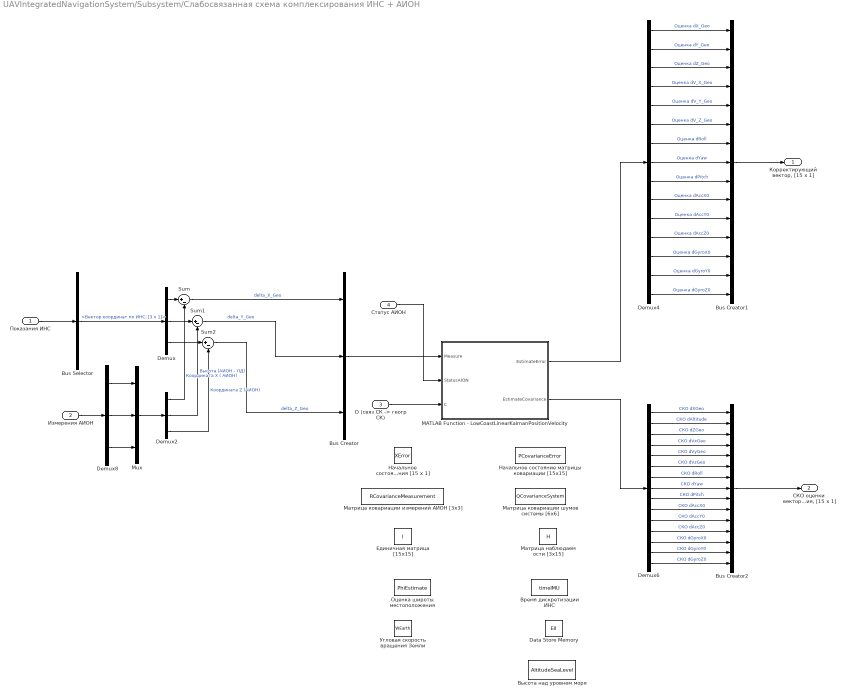
== system UAVIntegratedNavigationSystem/Subsystem/Слабосвязанная схема комплексирования ИНС + АИОН ==
  Показания ИНС : Inport
  Измерения АИОН : Inport  Port=2  SampleTime=0.1
  "D (связ СК -> геогр СК)" : Inport  Port=3
  Статус АИОН : Inport  Port=4
  Bus Creator : BusCreator  Inputs=3
  Bus Creator1 : BusCreator  Inputs=15
  Bus Creator2 : BusCreator  Inputs=15
  Bus Selector : BusSelector  OutputSignals=Вектор координат по ИНС; [3 x 1]
  Data Store Memory : DataStoreMemory  DataStoreName=Ell  ReadBeforeWriteMsg=warning  WriteAfterWriteMsg=warning  WriteAfterReadMsg=warning  InitialValue=[Ra;e]  ShowAdditionalParam=off  OutDataTypeStr=double
  Demux : Demux  Outputs=3
  Demux2 : Demux  Outputs=3
  Demux4 : Demux  Outputs=15
  Demux6 : Demux  Outputs=15
  Demux8 : Demux  Outputs=3
  MATLAB Function - LowCoastLinearKalmanPositionVelocity : MATLAB Function  TreatAsAtomicUnit=on
  Mux : Mux  Inputs=3
  Sum : Sum  Inputs=|+-
  Sum1 : Sum  Inputs=|+-
  Sum2 : Sum  Inputs=|+-
  Время дискретизации ИНС : DataStoreMemory  DataStoreName=timeIMU  ReadBeforeWriteMsg=warning  WriteAfterWriteMsg=warning  WriteAfterReadMsg=warning  InitialValue=1E-2  ShowAdditionalParam=off  OutDataTypeStr=double
  Высота над уровнем моря : DataStoreMemory  DataStoreName=AltitudeSeaLevel  ReadBeforeWriteMsg=warning  WriteAfterWriteMsg=warning  WriteAfterReadMsg=warning  InitialValue=H0  ShowAdditionalParam=off  OutDataTypeStr=double
  Единичная матрица [15x15] : DataStoreMemory  DataStoreName=I  ReadBeforeWriteMsg=warning  WriteAfterWriteMsg=warning  WriteAfterReadMsg=warning  InitialValue=eye(15)  ShowAdditionalParam=off  OutDataTypeStr=double
  Матрица ковариации измерений АИОН [3x3] : DataStoreMemory  DataStoreName=RCovarianceMeasurement  ReadBeforeWriteMsg=warning  WriteAfterWriteMsg=warning  WriteAfterReadMsg=warning  InitialValue=diag([ (0.1*SigmaAION)^2 (0.01*SigmaLaser)^2 (0.1*SigmaAION)^2 ])  ShowAdditionalParam=off  OutDataTypeStr=double
  Матрица ковариации шумов системы [6x6] : DataStoreMemory  DataStoreName=QCovarianceSystem  ReadBeforeWriteMsg=warning  WriteAfterWriteMsg=warning  WriteAfterReadMsg=warning  InitialValue=diag([SigmaAccel^2 SigmaAccel^2 SigmaAccel^2 SigmaGyro^2 SigmaGyro^2 SigmaGyro^2])  ShowAdditionalParam=off  OutDataTypeStr=double
  Матрица наблюдаемости [3x15] : DataStoreMemory  DataStoreName=H  ReadBeforeWriteMsg=warning  WriteAfterWriteMsg=warning  WriteAfterReadMsg=warning  InitialValue=[1 0 0 0 0 0 0 0 0 0 0 0 0 0 0;0 1 0 0 0 0 0 0 0 0 0 0 0 0 0; 0 0 1 0 0 0 0 0 0 0 0 0 0 0 0]  ShowAdditionalParam=off  OutDataTypeStr=double
  Начальное состояние вектора - состояния [15 x 1] : DataStoreMemory  DataStoreName=XError  ReadBeforeWriteMsg=warning  WriteAfterWriteMsg=warning  WriteAfterReadMsg=warning  InitialValue=[0;0;0;0;0;0;0;0;0;0;0;0;0;0;0]  ShowAdditionalParam=off  OutDataTypeStr=double
  Начальное состояние матрицы ковариации [15x15] : DataStoreMemory  DataStoreName=PCovarianceError  ReadBeforeWriteMsg=warning  WriteAfterWriteMsg=warning  WriteAfterReadMsg=warning  InitialValue=diag([10 10 10 2 2 2 1e-1 1e-1 1e-1 1e-3 1e-3 1e-3 1e-3 1e-3 1e-3])  ShowAdditionalParam=off  OutDataTypeStr=double
  Оценка широты местоположения : DataStoreMemory  DataStoreName=PhiEstimate  ReadBeforeWriteMsg=warning  WriteAfterWriteMsg=warning  WriteAfterReadMsg=warning  InitialValue=PhiInit  ShowAdditionalParam=off  OutDataTypeStr=double
  Угловая скорость вращения Земли : DataStoreMemory  DataStoreName=WEarth  ReadBeforeWriteMsg=warning  WriteAfterWriteMsg=warning  WriteAfterReadMsg=warning  InitialValue=WEarth  ShowAdditionalParam=off  OutDataTypeStr=double
  "Корректирующий вектор, [15 x 1]" : Outport
  "СКО оценки вектора состояния, [15 x 1]" : Outport  Port=2
  wires:
  Показания ИНС/1 -> Bus Selector/1
  Sum/1 -> Bus Creator/1  "delta_X_Geo"
  Sum1/1 -> Bus Creator/2  "delta_Y_Geo"
  Sum2/1 -> Bus Creator/3  "delta_Z_Geo"
  Bus Creator/1 -> MATLAB Function - LowCoastLinearKalmanPositionVelocity/1(Measure)
  MATLAB Function - LowCoastLinearKalmanPositionVelocity/1(EstimateError) -> Demux4/1
  Bus Creator1/1 -> "Корректирующий вектор, [15 x 1]"/1
  MATLAB Function - LowCoastLinearKalmanPositionVelocity/2(EstimateCovariance) -> Demux6/1
  Bus Selector/1 -> Demux/1  "<Вектор координат по ИНС; [3 x 1]>"
  Demux8/1 -> Mux/1
  Demux8/2 -> Mux/2
  Demux8/3 -> Mux/3
  Mux/1 -> Demux2/1
  Измерения АИОН/1 -> Demux8/1
  Статус АИОН/1 -> MATLAB Function - LowCoastLinearKalmanPositionVelocity/2(StatusAION)
  Demux6/1 -> Bus Creator2/1  "СКО dXGeo"
  Demux6/2 -> Bus Creator2/2  "СКО dAltitude"
  Demux6/3 -> Bus Creator2/3  "СКО dZGeo"
  Demux6/4 -> Bus Creator2/4  "СКО dVxGeo"
  Demux6/5 -> Bus Creator2/5  "СКО dVyGeo"
  Demux6/6 -> Bus Creator2/6  "СКО dVzGeo"
  Demux/1 -> Sum/1
  Demux2/1 -> Sum/2  "Координата X ( АИОН)"
  Demux/2 -> Sum1/1
  Demux2/2 -> Sum1/2  "Высота (АИОН - ЛД)"
  Demux2/3 -> Sum2/2  "Координата Z (АИОН)"
  Demux/3 -> Sum2/1
  Demux4/1 -> Bus Creator1/1  "Оценка dX_Geo"
  Demux4/2 -> Bus Creator1/2  "Оценка dY_Geo"
  Demux4/3 -> Bus Creator1/3  "Оценка dZ_Geo"
  Demux4/4 -> Bus Creator1/4  "Оценка dV_X_Geo"
  Demux4/5 -> Bus Creator1/5  "Оценка dV_Y_Geo"
  Demux4/6 -> Bus Creator1/6  "Оценка dV_Z_Geo"
  "D (связ СК -> геогр СК)"/1 -> MATLAB Function - LowCoastLinearKalmanPositionVelocity/3(C)
  Demux4/7 -> Bus Creator1/7  "Оценка dRoll"
  Demux4/8 -> Bus Creator1/8  "Оценка dYaw"
  Demux4/9 -> Bus Creator1/9  "Оценка dPitch"
  Demux6/7 -> Bus Creator2/7  "СКО dRoll"
  Demux6/8 -> Bus Creator2/8  "СКО dYaw"
  Demux6/9 -> Bus Creator2/9  "СКО dPitch"
  Bus Creator2/1 -> "СКО оценки вектора состояния, [15 x 1]"/1
  Demux6/10 -> Bus Creator2/10  "СКО dAccX0"
  Demux6/11 -> Bus Creator2/11  "СКО dAccY0"
  Demux6/12 -> Bus Creator2/12  "СКО dAccZ0"
  Demux6/13 -> Bus Creator2/13  "СКО dGyroX0"
  Demux6/14 -> Bus Creator2/14  "СКО dGyroY0"
  Demux6/15 -> Bus Creator2/15  "СКО dGyroZ0"
  Demux4/10 -> Bus Creator1/10  "Оценка dAccX0"
  Demux4/11 -> Bus Creator1/11  "Оценка dAccY0"
  Demux4/12 -> Bus Creator1/12  "Оценка dAccZ0"
  Demux4/13 -> Bus Creator1/13  "Оценка dGyroX0"
  Demux4/14 -> Bus Creator1/14  "Оценка dGyroY0"
  Demux4/15 -> Bus Creator1/15  "Оценка dGyroZ0"
